simulink model "list2_question2_simulink"  (R2014a)
settings: Solver=ode45  StartTime=0.0  StopTime=10.0  RelTol=1e-3
values from neighbouring files (symbols this model uses):
  B_J = 4    [list2_question2.m]
  G_J = 14400    [list2_question2.m]
  Kv = -1/3600 * 1.05    (= -0.000291666666667)    [list2_question2.m]
settings Model: Creator=Andre  LastModifiedBy=Andre
settings DataIOCC: SignalLoggingSaveFormat=ModelDataLogs
settings OptimizationCC: ExpressionDepthLimit=2147483647
settings DebuggingCC: UnderspecifiedInitializationDetection=Classic  FcnCallInpInsideContextMsg=UseLocalSettings  StateNameClashWarn=warning
settings GRTTargetCC: CombineOutputUpdateFcns=off  GRTInterface=on

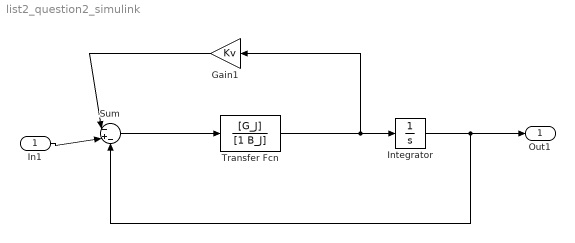
== system list2_question2_simulink ==
  In1 : Inport
  Gain1 : Gain  Gain=Kv
  Integrator : Integrator
  Sum : Sum  Inputs=|-+-
  Transfer Fcn : TransferFcn  Numerator=[G_J]  Denominator=[1 B_J]
  Out1 : Outport
  wires:
  Integrator/1 -> Out1/1, Sum/3
  Transfer Fcn/1 -> Integrator/1, Gain1/1
  Sum/1 -> Transfer Fcn/1
  In1/1 -> Sum/2
  Gain1/1 -> Sum/1
